simulink model "Hough_verify"  (R2013a)
settings: Solver=ode3  StartTime=0.0  StopTime=390  FixedStep=0.1  RelTol=1e-3
undefined symbols (not defined in the file): gray
libraries: visionsinks x1
settings Model: Creator=ZhaoJun  LastModifiedBy=ZhaoJun

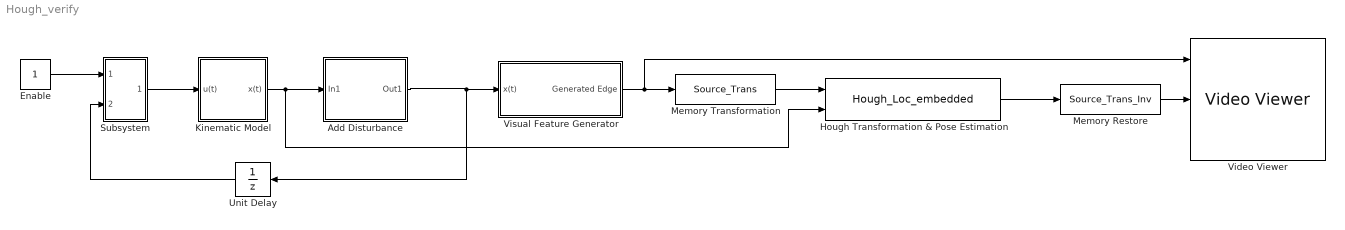
== system Hough_verify ==
  Add Disturbance : Subsystem
  Enable : Constant
  Hough Transformation & Pose Estimation : S-Function  FunctionName=Hough_Loc_embedded  EnableBusSupport=off
  Kinematic Model : Subsystem
  "Memory Restore " : S-Function  FunctionName=Source_Trans_Inv  EnableBusSupport=off
  Memory Transformation : S-Function  FunctionName=Source_Trans  EnableBusSupport=off
  Subsystem : Subsystem
  Unit Delay : UnitDelay  InitialCondition=[0 0 0]  SampleTime=-1
  Video Viewer : visionsinks/Video Viewer  inputType=Obsolete7b  imagePorts=Separate color signals  useColorMap=off  colormapValue=gray(256)  specRange=off  minInputVal=0  maxInputVal=255  FigPos=[1 1038 1920 938]  AxisZoom=on  trueSizedOnce=off  OpenAtMdlStart=on  DefaultConfigurationName=vipscopes.VideoViewerScopeCfg
  Visual Feature Generator : Subsystem
  wires:
  Hough Transformation & Pose Estimation/2 -> "Memory Restore "/1
  Memory Transformation/1 -> Hough Transformation & Pose Estimation/1
  "Memory Restore "/1 -> Video Viewer/2
  Add Disturbance/1(Out1) -> Visual Feature Generator/1(x(t)), Unit Delay/1
  Enable/1 -> Subsystem/1(Enable)
  Unit Delay/1 -> Subsystem/2(x(t-1))
  Kinematic Model/1(x(t)) -> Hough Transformation & Pose Estimation/2, Add Disturbance/1(In1)
  Subsystem/1(u(t)) -> Kinematic Model/1(u(t))
  Visual Feature Generator/1(Generated Edge) -> Memory Transformation/1, Video Viewer/1

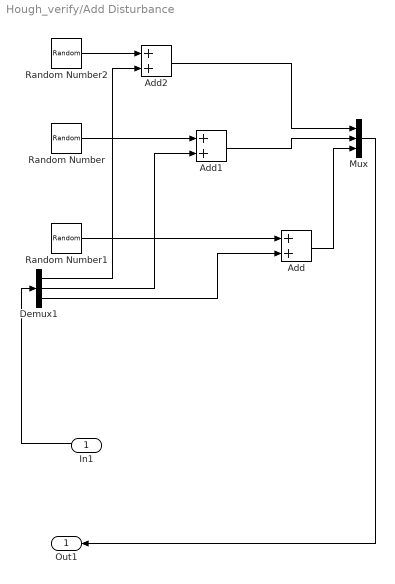
== system Hough_verify/Add Disturbance ==
  In1 : Inport
  Add : Sum
  Add1 : Sum
  Add2 : Sum
  Demux1 : Demux  Outputs=3
  Mux : Mux  Inputs=3
  Random Number : RandomNumber  Variance=0.00027778  Seed=3
  Random Number1 : RandomNumber  Variance=0.0016
  Random Number2 : RandomNumber  Variance=0.00027778  Seed=5
  Out1 : Outport
  wires:
  Random Number2/1 -> Add2/1
  Demux1/1 -> Add2/2
  Random Number/1 -> Add1/1
  Demux1/2 -> Add1/2
  Demux1/3 -> Add/2
  Random Number1/1 -> Add/1
  Add2/1 -> Mux/1
  Add1/1 -> Mux/2
  Add/1 -> Mux/3
  Mux/1 -> Out1/1
  In1/1 -> Demux1/1

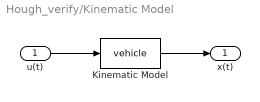
== system Hough_verify/Kinematic Model ==
  u(t) : Inport
  Kinematic Model : S-Function  FunctionName=vehicle  Parameters=0,0,0  EnableBusSupport=off
  x(t) : Outport
  wires:
  u(t)/1 -> Kinematic Model/1
  Kinematic Model/1 -> x(t)/1

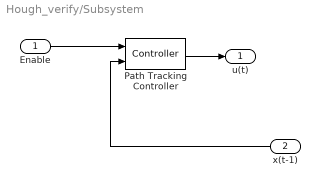
== system Hough_verify/Subsystem ==
  Enable : Inport
  x(t-1) : Inport  Port=2
  Path Tracking Controller : S-Function  FunctionName=Controller  EnableBusSupport=off
  u(t) : Outport
  wires:
  x(t-1)/1 -> Path Tracking Controller/2
  Enable/1 -> Path Tracking Controller/1
  Path Tracking Controller/1 -> u(t)/1

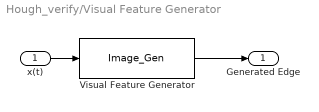
== system Hough_verify/Visual Feature Generator ==
  x(t) : Inport
  Visual Feature Generator : S-Function  FunctionName=Image_Gen  EnableBusSupport=off
  Generated Edge : Outport
  wires:
  x(t)/1 -> Visual Feature Generator/1
  Visual Feature Generator/1 -> Generated Edge/1
